simulink model "THIPWM"  (R2019a)
settings: Solver=VariableStepAuto  StartTime=0.0  StopTime=0.5  MinStep=1e-5  RelTol=1e-3
libraries: simulink x3, powerlib_meascontrol x1
settings Model: Creator=Amanna  LastModifiedBy=Amanna

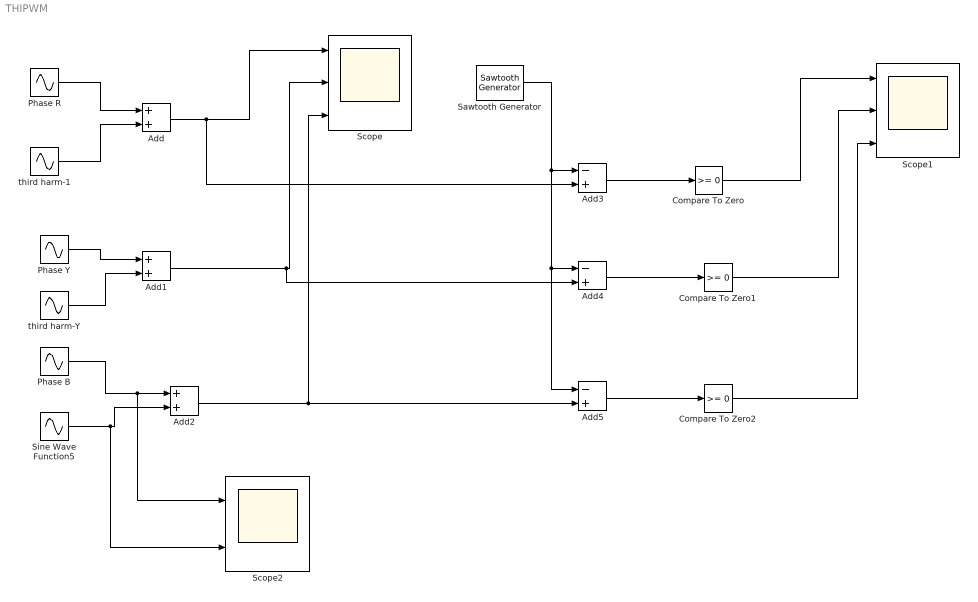
== system THIPWM ==
  Add : Sum
  Add1 : Sum
  Add2 : Sum
  Add3 : Sum  Inputs=-+
  Add4 : Sum  Inputs=-+
  Add5 : Sum  Inputs=-+
  Compare To Zero : simulink/Logic and Bit Operations/Compare To Zero  relop=>=  OutDataTypeStr=boolean
  Compare To Zero1 : simulink/Logic and Bit Operations/Compare To Zero  relop=>=  OutDataTypeStr=boolean
  Compare To Zero2 : simulink/Logic and Bit Operations/Compare To Zero  relop=>=  OutDataTypeStr=boolean
  Phase B : Sin  Amplitude=1.1547  Frequency=2*pi*50  Phase=4*pi/3  SampleTime=0
  "Phase R " : Sin  Amplitude=1.1547  Frequency=2*pi*50  SampleTime=0
  Phase Y : Sin  Amplitude=1.1547  Frequency=2*pi*50  Phase=2*pi/3  SampleTime=0
  Sawtooth Generator : powerlib_meascontrol/Pulse & Signal Generators/Sawtooth Generator  Freq=2  Phase=180  Ts=0
      settings: SourceProductName=Simscape Electrical
  Scope : Scope  NumInputPorts=3
  Scope1 : Scope  NumInputPorts=3
  Scope2 : Scope  NumInputPorts=2
  Sine Wave Function5 : Sin  Amplitude=0.193  Frequency=2*pi*50*3  SampleTime=0
  third harm-1 : Sin  Amplitude=0.193  Frequency=2*pi*50*3  SampleTime=0
  third harm-Y : Sin  Amplitude=0.193  Frequency=2*pi*50*3  SampleTime=0
  wires:
  "Phase R "/1 -> Add/1
  third harm-1/1 -> Add/2
  Phase Y/1 -> Add1/1
  third harm-Y/1 -> Add1/2
  Phase B/1 -> Scope2/1, Add2/1
  Sine Wave Function5/1 -> Scope2/2, Add2/2
  Add/1 -> Add3/2, Scope/1
  Add1/1 -> Add4/2, Scope/2
  Add2/1 -> Add5/2, Scope/3
  Sawtooth Generator/1 -> Add5/1, Add4/1, Add3/1
  Add3/1 -> Compare To Zero/1
  Add4/1 -> Compare To Zero1/1
  Add5/1 -> Compare To Zero2/1
  Compare To Zero/1 -> Scope1/1
  Compare To Zero1/1 -> Scope1/2
  Compare To Zero2/1 -> Scope1/3
